simulink model "RealniSistem"  (R2020b)
settings: Solver=VariableStepAuto  StartTime=0.0  StopTime=140  RelTol=1e-3
libraries: PoKeysIOInterface x1, powerlib_meascontrol x1
settings Model: Creator=64210381  LastModifiedBy=64210381

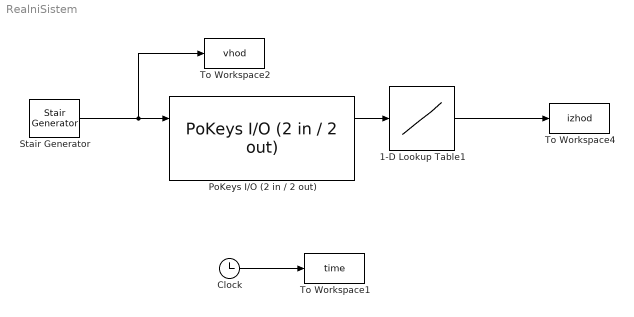
== system RealniSistem ==
  1-D Lookup Table1 : Lookup_n-D  NumberOfTableDimensions=1  BreakpointsForDimension1=[0.83, 3.52, 6]  Table=[177, 90, 14]  SampleTime=0.1  InternalRulePriority=Speed  RndMeth=Simplest  InputSameDT=on
  Clock : Clock
  PoKeys I/O (2 in / 2 out) : PoKeysIOInterface/PoKeys I//O (2 in // 2 out)  MaxPowerLimit=100.0  IOTs=0.002  IOSerial=507
      settings: SourceProductName=PoKeys I/O interface
  Stair Generator : powerlib_meascontrol/Pulse & Signal Generators/Stair Generator  t=0:20:100  e=5:0.5:7.5  Ts=0
  To Workspace1 : ToWorkspace  VariableName=time  SampleTime=-1
  To Workspace2 : ToWorkspace  VariableName=vhod  SampleTime=-1
  To Workspace4 : ToWorkspace  VariableName=izhod  SaveFormat=Timeseries  SampleTime=0.1
  wires:
  Stair Generator/1 -> PoKeys I/O (2 in / 2 out)/1, To Workspace2/1
  Clock/1 -> To Workspace1/1
  1-D Lookup Table1/1 -> To Workspace4/1
  PoKeys I/O (2 in / 2 out)/1 -> 1-D Lookup Table1/1
